simulink model "bmm_sim"  (R2021b)
settings: Solver=FixedStepAuto  StartTime=0.0  StopTime=180  FixedStep=1  RelTol=1e-3
settings Model: Creator=marek  LastModifiedBy=marekwadinger
settings DataIOCC: ExternalInput=tt

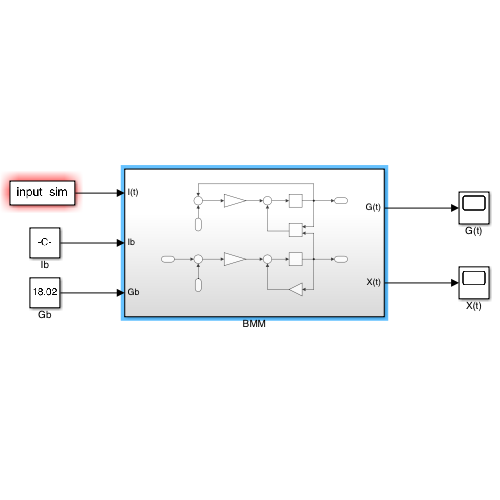
[thumbnail: Simulink's stored preview of the top-level diagram]
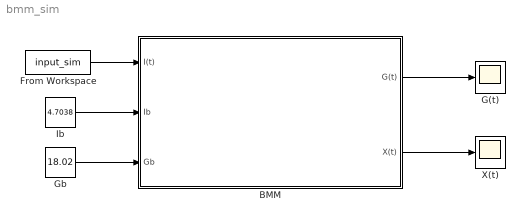
== system bmm_sim ==
  BMM : Subsystem
  From Workspace : FromWorkspace  VariableName=input_sim
  G(t) : Scope
  Gb : Constant  Value=18.02  SampleTime=0
  Ib : Constant  Value=4.7038  SampleTime=0
  X(t) : Scope
  wires:
  Ib/1 -> BMM/2(Ib)
  Gb/1 -> BMM/3(Gb)
  BMM/2(X(t)) -> X(t)/1
  From Workspace/1 -> BMM/1(I(t))
  BMM/1(G(t)) -> G(t)/1

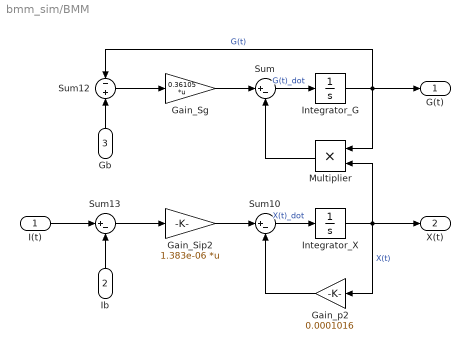
== system bmm_sim/BMM ==
  I(t) : Inport
  Ib : Inport  Port=2
  Gb : Inport  Port=3
  Gain_Sg : Gain  Gain=0.36105  Multiplication=Matrix(K*u)
  Gain_Sip2 : Gain  Gain=1.383e-06  Multiplication=Matrix(K*u)
  Gain_p2 : Gain  Gain=0.0001016
  Integrator_G : Integrator  InitialCondition=16  LimitOutput=on  UpperSaturationLimit=100
  Integrator_X : Integrator
  Multiplier : Product
  Sum : Sum  Inputs=|+-
  Sum10 : Sum  Inputs=|+-
  Sum12 : Sum  Inputs=-|+
  Sum13 : Sum  Inputs=|+-
  G(t) : Outport
  X(t) : Outport  Port=2
  wires:
  Integrator_X/1 -> X(t)/1, Multiplier/2, Gain_p2/1  "X(t)"
  Sum13/1 -> Gain_Sip2/1
  Gain_Sip2/1 -> Sum10/1
  I(t)/1 -> Sum13/1
  Ib/1 -> Sum13/2
  Gb/1 -> Sum12/2
  Sum12/1 -> Gain_Sg/1
  Gain_Sg/1 -> Sum/1
  Multiplier/1 -> Sum/2
  Sum/1 -> Integrator_G/1  "G(t)_dot"
  Sum10/1 -> Integrator_X/1  "X(t)_dot"
  Gain_p2/1 -> Sum10/2
  Integrator_G/1 -> Sum12/1, Multiplier/1, G(t)/1  "G(t)"
